simulink model "motor_ideal"  (R2023b)
settings: Solver=VariableStepAuto  StartTime=0.0  StopTime=5  RelTol=1e-3
undefined symbols (not defined in the file): ke, p, voltage
settings Model: Creator=miqui  LastModifiedBy=miqui

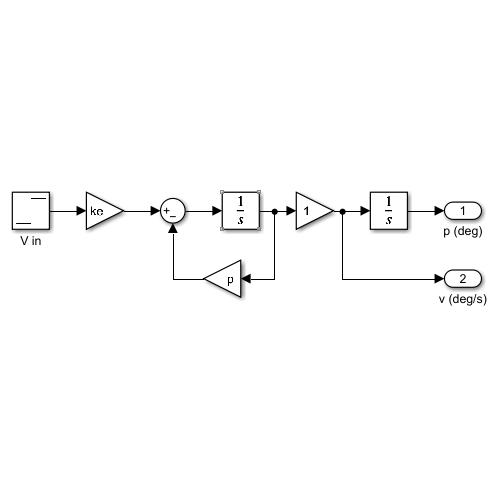
[thumbnail: Simulink's stored preview of the top-level diagram]
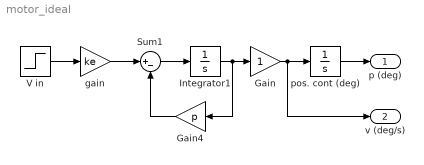
== system motor_ideal ==
  Gain : Gain
  Gain4 : Gain  Gain=p
  Integrator1 : Integrator
  Sum1 : Sum  Inputs=|+-
  V in : Step  After=voltage  SampleTime=0
  gain : Gain  Gain=ke
  pos. cont (deg) : Integrator
  p (deg) : Outport
  v (deg/s) : Outport  Port=2
  wires:
  Gain/1 -> pos. cont (deg)/1, v (deg/s)/1
  gain/1 -> Sum1/1
  Gain4/1 -> Sum1/2
  pos. cont (deg)/1 -> p (deg)/1
  Sum1/1 -> Integrator1/1
  Integrator1/1 -> Gain/1, Gain4/1
  V in/1 -> gain/1
